simulink model "no_chattering"  (Simulink 7.7)
settings: Solver=ode45  StartTime=0.0  StopTime=20  RelTol=1e-3
values from neighbouring files (symbols this model uses):
  k1 = 1/yl    (= 2.5)    [Laboratorio2.m]
  k2 = sqrt(2*k1)    [Laboratorio2.m]
  pos0 = 10    [Laboratorio2.m]
  yl = 0.4    [Laboratorio2.m]
libraries: simulink x1
settings Model: Creator=g  LastModifiedBy=g
settings DebuggingCC: SolverPrmCheckMsg=none

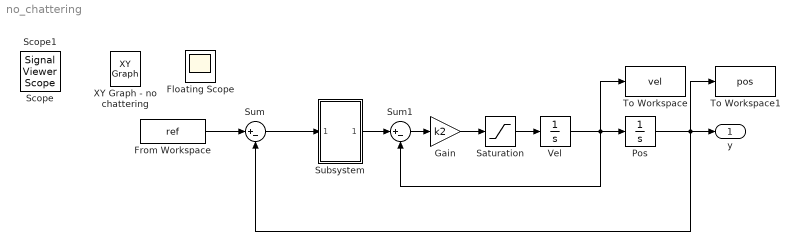
== system no_chattering ==
  From Workspace : FromWorkspace  VariableName=ref  SampleTime=0  OutputAfterFinalValue=Holding final value
  Gain : Gain  Gain=k2
  Pos : Integrator  InitialCondition=pos0
  Saturation : Saturate  UpperLimit=1  LowerLimit=-1
  Subsystem : Subsystem
  Sum : Sum  Inputs=|+-
  Sum1 : Sum  Inputs=|+-
  To Workspace : ToWorkspace  VariableName=vel  SampleTime=-1  SaveFormat=Array
  To Workspace1 : ToWorkspace  VariableName=pos  SampleTime=-1  SaveFormat=Array
  Vel : Integrator
  y : Outport
  Floating Scope : Scope
      settings: Floating=on
  Scope : SignalViewerScope  IOType=viewer  RefreshTime=0.035000
  Scope1 : SignalViewerScope  IOType=viewer  RefreshTime=0.035000
  XY Graph - no chattering : simulink/Sinks/XY Graph  IOType=viewer  SystemSampleTime=-1  xmin=xmin  xmax=xmax  ymin=ymin  ymax=ymax  st=-1
  wires:
  Pos/1 -> Sum/2, To Workspace1/1, y/1
  Vel/1 -> Sum1/2, Pos/1, To Workspace/1
  Sum/1 -> Subsystem/1(In1)
  Subsystem/1(Out1) -> Sum1/1
  Sum1/1 -> Gain/1
  Gain/1 -> Saturation/1
  Saturation/1 -> Vel/1
  From Workspace/1 -> Sum/1

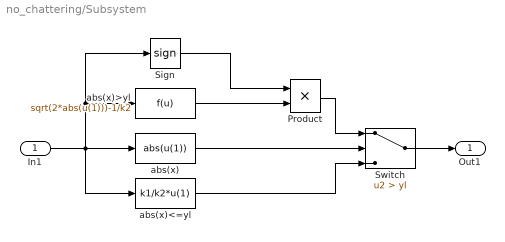
== system no_chattering/Subsystem ==
  In1 : Inport
  Product : Product  RndMeth=Zero
  Sign : Signum
  Switch : Switch  Criteria=u2 > Threshold  Threshold=yl
  abs(x) : Fcn  Expr=abs(u(1))
  abs(x)<=yl : Fcn  Expr=k1/k2*u(1)
  abs(x)>yl : Fcn  Expr=sqrt(2*abs(u(1)))-1/k2
  Out1 : Outport
  wires:
  In1/1 -> abs(x)<=yl/1, abs(x)>yl/1, Sign/1, abs(x)/1
  abs(x)<=yl/1 -> Switch/3
  Switch/1 -> Out1/1
  abs(x)/1 -> Switch/2
  Product/1 -> Switch/1
  abs(x)>yl/1 -> Product/2
  Sign/1 -> Product/1
